simulink model "PPS_Radar"  (Simulink 7.6)
settings: Solver=FixedStepDiscrete  SolverMode=SingleTasking  StartTime=0.0  StopTime=inf  FixedStep=0.01  RelTol=1e-3
settings Model: Creator=Krzysztof  LastModifiedBy=pastora
settings DataIOCC: LimitDataPoints=off  MaxDataPoints=1  SaveOutput=off  DSMLogging=off  InspectSignalLogs=on
settings OptimizationCC: InlineParams=on
settings DebuggingCC: UnknownTsInhSupMsg=none
settings ModelReferenceCC: ModelReferenceNumInstancesAllowed=Single

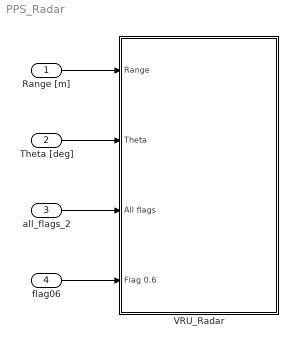
== system PPS_Radar ==
  Range [m] : Inport
  Theta [deg] : Inport  Port=2
  all_flags_2 : Inport  Port=3
  flag06 : Inport  Port=4
  VRU_Radar : Subsystem  mask{mfreq=100, dfreq=25, TISdet=32}
      mask prompts: mfreq "Model frequency [Hz]"; dfreq "Display frequency [Hz]"; TISdet "Max. number of detected objects [-]"
  wires:
  Range [m]/1 -> VRU_Radar/1(Range)
  Theta [deg]/1 -> VRU_Radar/2(Theta)
  all_flags_2/1 -> VRU_Radar/3(All flags)
  flag06/1 -> VRU_Radar/4(Flag 0.6)

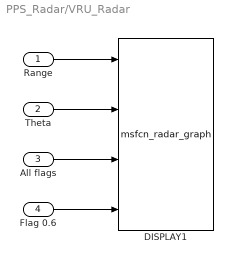
== system PPS_Radar/VRU_Radar ==
  Range : Inport
  Theta : Inport  Port=2
  All flags : Inport  Port=3  OutDataTypeStr=boolean
  Flag 0.6 : Inport  Port=4  OutDataTypeStr=boolean
  DISPLAY1 : M-S-Function  FunctionName=msfcn_radar_graph  Parameters=dfreq TISdet
  wires:
  Range/1 -> DISPLAY1/1
  Theta/1 -> DISPLAY1/2
  All flags/1 -> DISPLAY1/3
  Flag 0.6/1 -> DISPLAY1/4
